simulink model "CurveTracking"  (R2020a)
settings: Solver=VariableStepAuto  StartTime=0.0  StopTime=10  RelTol=1e-3
values from neighbouring files (symbols this model uses):
  goalRadius = 0.1    [main.m]
  lookaheadDist = 0.001    [main.m]
  maxLinearVelocity = 80    [main.m]
  path = randomcurve(100,75)    [main.m]    (also in randomcurve.m = cumsum(step))
  sampleTime = 0.01    [main.m]
  state_0 = [0 0 0]    [main.m]
  wheelBase = 1    [main.m]
undefined symbols (not defined in the file or in its folder): DiscIntNeverNeededParam
libraries: robotalgslib x1
settings Model: Creator=William  LastModifiedBy=William
settings DataIOCC: ReturnWorkspaceOutputs=off

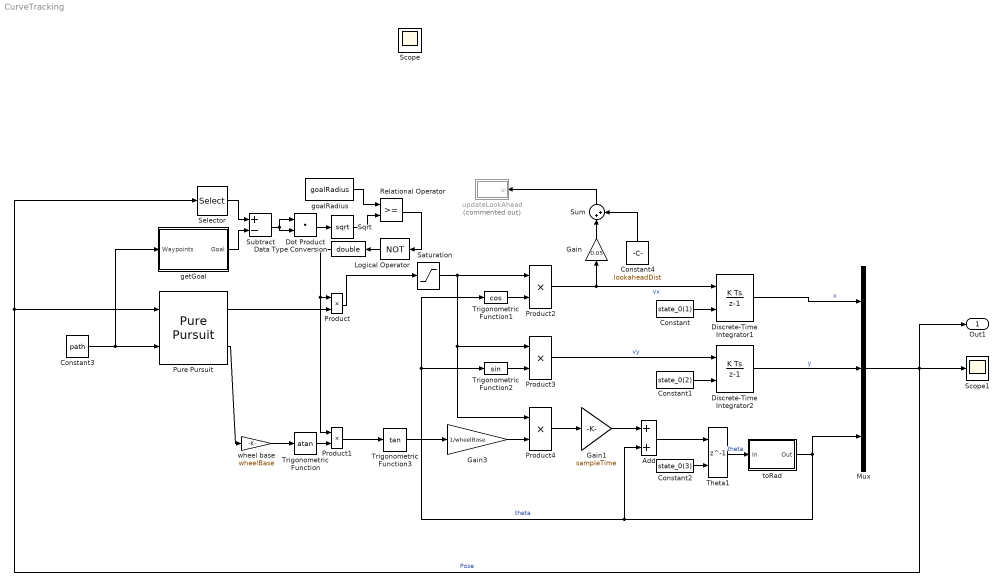
== system CurveTracking ==
  " getGoal" : MATLAB Function  TreatAsAtomicUnit=on
  Add : Sum
  Constant : Constant  Value=state_0(1)
  Constant1 : Constant  Value=state_0(2)
  Constant2 : Constant  Value=state_0(3)
  Constant3 : Constant  Value=path
  Constant4 : Constant  Value=lookaheadDist
  Data Type Conversion : DataTypeConversion  OutDataTypeStr=double
  Discrete-Time Integrator1 : DiscreteIntegrator  InitialConditionSource=external  SampleTime=sampleTime  ICPrevOutput=DiscIntNeverNeededParam  ICPrevScaledInput=DiscIntNeverNeededParam
  Discrete-Time Integrator2 : DiscreteIntegrator  InitialConditionSource=external  SampleTime=sampleTime  ICPrevOutput=DiscIntNeverNeededParam  ICPrevScaledInput=DiscIntNeverNeededParam
  Dot Product : DotProduct  InputSameDT=on  OutDataTypeStr=Inherit: Inherit via internal rule
  Gain : Gain  Gain=0.05
  Gain1 : Gain  Gain=sampleTime
  Gain3 : Gain  Gain=1/wheelBase
  Logical Operator : Logic  Operator=NOT  AllPortsSameDT=off  OutDataTypeStr=boolean
  Mux : Mux  Inputs=3
  Product{,1..4} (5 alike) : Product
  Pure Pursuit : robotalgslib/Pure Pursuit  DesiredLinearVelocity=desiredLinearVelocity  MaxAngularVelocity=maxAngularVelocity  LookaheadDistance=lookaheadDist  TargetDirPort=off  SimulateUsing=Code generation
  Relational Operator : RelationalOperator  OutDataTypeStr=boolean  RndMeth=Simplest
  Saturation : Saturate  UpperLimit=maxLinearVelocity  LowerLimit=-maxLinearVelocity
  Scope1 : Scope
  Selector : Selector  InputPortWidth=3  IndexOptions=Index vector (dialog)  Indices=[1 2]  OutputSizes=1
  Sqrt : Sqrt  SaturateOnIntegerOverflow=on
  Subtract : Sum  Inputs=+-
  Sum : Sum  Inputs=|++
  Theta1 : Delay  DelayLength=1  InitialConditionSource=Input port
      settings: InputPortMap=u0,p4
  Trigonometric Function : Trigonometry  Operator=atan
  Trigonometric Function1 : Trigonometry  Operator=cos
  Trigonometric Function2 : Trigonometry
  Trigonometric Function3 : Trigonometry  Operator=tan
  goalRadius : Constant  Value=goalRadius
  toRad : MATLAB Function  TreatAsAtomicUnit=on
      settings: CopyFcn=set_param(gcbh,'LinkStatus','none');
  updateLookAhead : MATLAB Function  Commented=on  TreatAsAtomicUnit=on
  wheel base : Gain  Gain=wheelBase
  Out1 : Outport  SampleTime=sampleTime
  Scope : Scope
  wires:
  Constant3/1 -> " getGoal"/1(Waypoints), Pure Pursuit/2
  " getGoal"/1(Goal) -> Subtract/2
  Selector/1 -> Subtract/1
  Subtract/1 -> Dot Product/2, Dot Product/1
  Dot Product/1 -> Sqrt/1
  goalRadius/1 -> Relational Operator/1
  Sqrt/1 -> Relational Operator/2
  Relational Operator/1 -> Logical Operator/1
  Logical Operator/1 -> Data Type Conversion/1
  Data Type Conversion/1 -> Product1/1, Product/1
  Pure Pursuit/1 -> Product/2
  Pure Pursuit/2 -> wheel base/1
  wheel base/1 -> Trigonometric Function/1
  Trigonometric Function/1 -> Product1/2
  Product/1 -> Saturation/1
  Saturation/1 -> Product4/1, Product3/1, Product2/1
  Trigonometric Function1/1 -> Product2/2
  Product1/1 -> Trigonometric Function3/1
  Trigonometric Function3/1 -> Gain3/1
  Gain3/1 -> Product4/2
  Product4/1 -> Gain1/1
  Gain1/1 -> Add/1
  Constant2/1 -> Theta1/2
  Add/1 -> Theta1/1
  Theta1/1 -> toRad/1(In)  "theta"
  toRad/1(Out) -> Add/2, Trigonometric Function1/1, Trigonometric Function2/1, Mux/3  "theta"
  Product2/1 -> Discrete-Time Integrator1/1, Gain/1  "vx"
  Constant/1 -> Discrete-Time Integrator1/2
  Product3/1 -> Discrete-Time Integrator2/1  "vy"
  Constant1/1 -> Discrete-Time Integrator2/2
  Discrete-Time Integrator1/1 -> Mux/1  "x"
  Discrete-Time Integrator2/1 -> Mux/2  "y"
  Mux/1 -> Out1/1, Scope1/1, Pure Pursuit/1, Selector/1  "Pose"
  Trigonometric Function2/1 -> Product3/2
  Constant4/1 -> Sum/2
  Gain/1 -> Sum/1
  Sum/1 -> updateLookAhead/1(u)

== matlab function CurveTracking/updateLookAhead ==
  data: u input
function updateLookAhead(u)
    coder.extrinsic('set_param');
    set_param('CurveTracking/Pure Pursuit','LookaheadDistance',u);

== matlab function CurveTracking/toRad ==
  data: In input; Out output
function Out = toRad(In)
%#codegen
Out = angdiff(0*In, In);

== matlab function CurveTracking/ getGoal ==
  data: Waypoints input; Goal output size=[2 1]
function Goal = getGoal(Waypoints)
%#codegen
b = isnan(Waypoints);
[rows,~] = find(b);
ridx = setdiff(1:size(Waypoints,1), sort(rows));
Goal = [Waypoints(ridx(end), 1) Waypoints(ridx(end), 2)]';
